simulink model "Lab2_Pole_Placement_Continuous"  (R2017b)
settings: Solver=VariableStepAuto  StartTime=0.0  StopTime=2  RelTol=1e-3
values from neighbouring files (symbols this model uses):
  f0 = F(2)    [Lab2_Pole_Placement.m]
  f1 = F(1)    [Lab2_Pole_Placement.m]
  g0 = F(4)    [Lab2_Pole_Placement.m]
  g1 = F(3)    [Lab2_Pole_Placement.m]
  K1 = 0.66538    [Lab2.m]    (also in Lab2_Pole_Placement.m)
  Kp = 15    [Lab2.m]    (also in Lab2_Pole_Placement.m = 1)
  tau = 0.030541    [Lab2.m]    (also in Lab2_Pole_Placement.m)
settings Model: Creator=jrampert  LastModifiedBy=joe
settings CodeAppCC: StateflowObjectComments=on

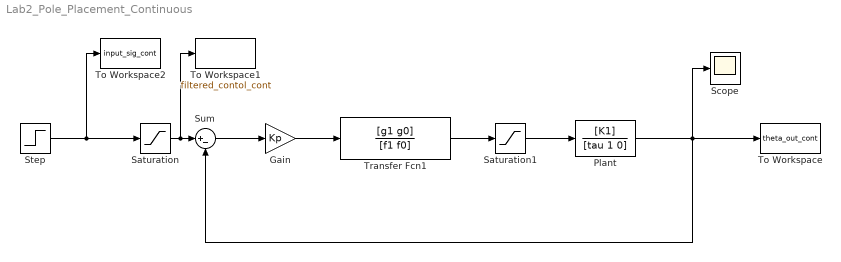
== system Lab2_Pole_Placement_Continuous ==
  Gain : Gain  Gain=Kp
  Plant : TransferFcn  Numerator=[K1]  Denominator=[tau 1 0]
  Saturation : Saturate  UpperLimit=0.785  LowerLimit=-0.785
  Saturation1 : Saturate  UpperLimit=6  LowerLimit=-6
  Scope : Scope
  Step : Step  Before=-0.7  After=0.7  SampleTime=0
  Sum : Sum  Inputs=|+-
  To Workspace : ToWorkspace  VariableName=theta_out_cont  SaveFormat=Timeseries  SampleTime=-1
  To Workspace1 : ToWorkspace  VariableName=filtered_contol_cont  SaveFormat=Timeseries  SampleTime=-1
  To Workspace2 : ToWorkspace  VariableName=input_sig_cont  SaveFormat=Timeseries  SampleTime=-1
  Transfer Fcn1 : TransferFcn  Numerator=[g1 g0]  Denominator=[f1 f0]
  wires:
  Saturation/1 -> To Workspace1/1, Sum/1
  Plant/1 -> Scope/1, Sum/2, To Workspace/1
  Step/1 -> To Workspace2/1, Saturation/1
  Saturation1/1 -> Plant/1
  Transfer Fcn1/1 -> Saturation1/1
  Sum/1 -> Gain/1
  Gain/1 -> Transfer Fcn1/1
